simulink model "Aufgabe2"  (R2015b)
settings: Solver=VariableStepAuto  StartTime=0.0  StopTime=10  RelTol=1e-3
InitFcn:
  | Aufgabe2_calc
values from neighbouring files (symbols this model uses):
  R1 = U/ I    (= 10000)    [Aufgabe2_calc.m]    (also in Aufgabe3_calc.m = 0.1)
  tau = 1.5    [Aufgabe2_calc.m]
libraries: fl_lib x5, nesl_utility x2
settings Model: Creator=lukaskiechle  LastModifiedBy=lukaskiechle

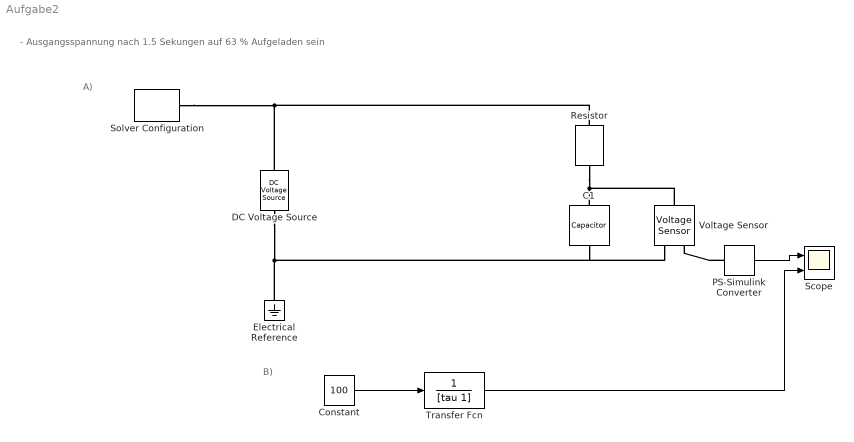
== system Aufgabe2 ==
  note: A)
  note: - Ausgangsspannung nach 1.5 Sekungen auf 63 % Aufgeladen sein
  note: B)
  C1 : fl_lib/Electrical/Electrical Elements/Capacitor  c=C1 F  r=0 Ohm  g=0 1/Ohm  i_specify=off  i_priority=None  i=0 A  v_specify=off  v_priority=None  v=0 V  vc_specify=off  vc_priority=None  vc=0 V
  Constant : Constant  Value=100
  DC Voltage Source : fl_lib/Electrical/Electrical Sources/DC Voltage Source  v0=100 V
  Electrical Reference : fl_lib/Electrical/Electrical Elements/Electrical Reference
  PS-Simulink Converter : nesl_utility/PS-Simulink Converter  PhysicalDomain=network_engine_domain  SubClassName=ps_output  LeftPortType=input  RightPortType=output  PseudoPeriodic=off  Frequencies=[]  Unit=V  AffineConversion=off
  Resistor : fl_lib/Electrical/Electrical Elements/Resistor  R=R1 Ohm  i_specify=off  i_priority=None  i=0 A  v_specify=off  v_priority=None  v=0 V
  Scope : Scope  NumInputPorts=2
  Solver Configuration : nesl_utility/Solver Configuration  PhysicalDomain=network_engine_domain  SubClassName=solver  LeftPortType=input  RightPortType=generic  Accelerate=off  Tones=[]  Harmonics=[]  SimulateNoise=off  Profile=off  UseLocalSampling=off  EnableSwitchedLinearOptims=on  FrequencyDomain=off  UseCCode=off  RelTol=0.001  AbsTol=1e-06  MinStep=1e-09  ToWorkspace=off  RevertToSquareIcSolve=off  NumHomotopyIterations=100  PhasorMode=off  PhasorModeNumHarmonics=1  DoDC=off  ResidualTolerance=1e-09  UseLocalSolver=off  LocalSolverChoice=NE_BACKWARD_EULER_ADVANCER  LocalSolverSampleTime=0.001  DoFixedCost=off  MaxNonlinIter=3  MaxModeIter=2  LinearAlgebra=Sparse  DelaysMemoryBudget=1024  AutomaticFiltering=on  FilteringTimeConstant=0.001
  Transfer Fcn : TransferFcn  Denominator=[tau 1]
  Voltage Sensor : fl_lib/Electrical/Electrical Sensors/Voltage Sensor
  wires:
  PS-Simulink Converter/1 -> Scope/1
  Constant/1 -> Transfer Fcn/1
  Transfer Fcn/1 -> Scope/2
  connections:
  Solver Configuration/RConn1 -- Resistor/LConn1 -- DC Voltage Source/LConn1
  Voltage Sensor/LConn1 -- Resistor/RConn1 -- C1/LConn1
  Electrical Reference/LConn1 -- DC Voltage Source/RConn1 -- C1/RConn1 -- Voltage Sensor/RConn2
  PS-Simulink Converter/LConn1 -- Voltage Sensor/RConn1
